simulink model "motorsim"  (R2021b)
settings: Solver=VariableStepAuto  StartTime=0.0  StopTime=10.0  RelTol=1e-3
values from neighbouring files (symbols this model uses):
  b = 0.5    [Assignment2_Curtis.m]    (also in Assignment2m_Curtis.m)
  J = 0.05    [Assignment2_Curtis.m]    (also in Assignment2m_Curtis.m)
  Ke = 0.5    [Assignment2_Curtis.m]    (also in Assignment2m_Curtis.m)
  Kt = 0.5    [Assignment2_Curtis.m]    (also in Assignment2m_Curtis.m)
  Ra = 1    [Assignment2_Curtis.m]    (also in Assignment2m_Curtis.m)
settings Model: Creator=Alex  LastModifiedBy=Alex

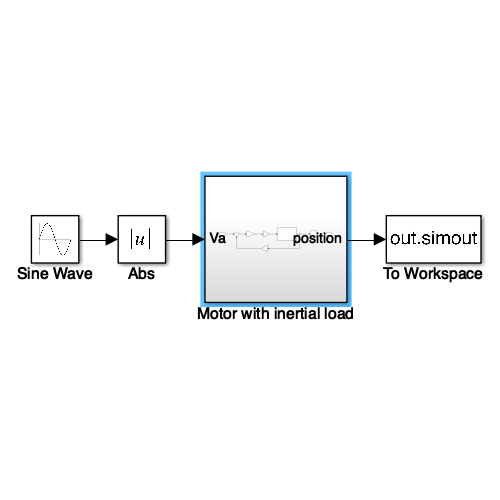
[thumbnail: Simulink's stored preview of the top-level diagram]
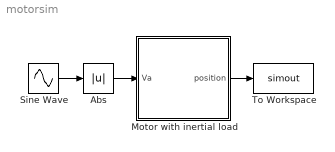
== system motorsim ==
  Abs : Abs
  Motor with inertial load : Subsystem
  Sine Wave : Sin  SampleTime=0
  To Workspace : ToWorkspace  VariableName=simout  SaveFormat=Timeseries  SampleTime=-1
  wires:
  Sine Wave/1 -> Abs/1
  Abs/1 -> Motor with inertial load/1(Va)
  Motor with inertial load/1(position) -> To Workspace/1

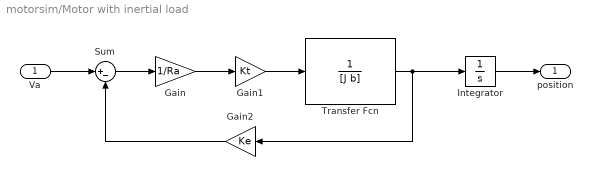
== system motorsim/Motor with inertial load ==
  Va : Inport
  Gain : Gain  Gain=1/Ra
  Gain1 : Gain  Gain=Kt
  Gain2 : Gain  Gain=Ke
  Integrator : Integrator
  Sum : Sum  Inputs=|+-
  Transfer Fcn : TransferFcn  Denominator=[J b]
  position : Outport
  wires:
  Va/1 -> Sum/1
  Integrator/1 -> position/1
  Sum/1 -> Gain/1
  Gain/1 -> Gain1/1
  Gain2/1 -> Sum/2
  Transfer Fcn/1 -> Integrator/1, Gain2/1
  Gain1/1 -> Transfer Fcn/1
